simulink model "ACFT_cae"  (R2024a)
settings: Solver=ode4  StartTime=0.0  StopTime=10.0  FixedStep=0.01  RelTol=1e-3  EnableMultiTasking=on
values from neighbouring files (symbols this model uses):
  Inertia = [Ixx 0 0; 0 Iyy 0; 0 0 Izz]    [Initialization.m]    (also in Initialization_alt2.m; Initialization_cg1.m; Initialization_loop.m; Initialization_v2.m)
libraries: AerodynamicModel x1, AtmosphericModel x1, EqM x1, Propulsion x1
settings Model: Creator=Caê  LastModifiedBy=Caê
settings RTWCC: GPUComputeCapability=3.5

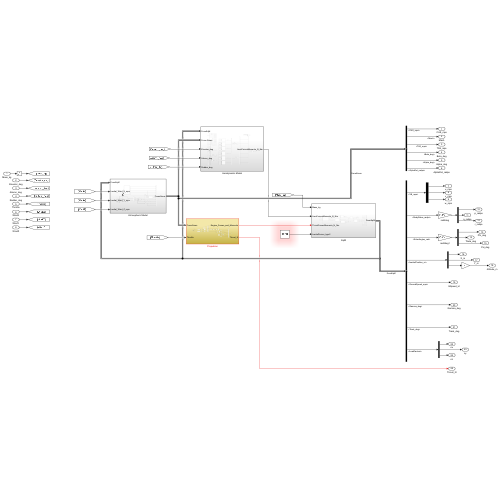
[thumbnail: Simulink's stored preview of the top-level diagram]
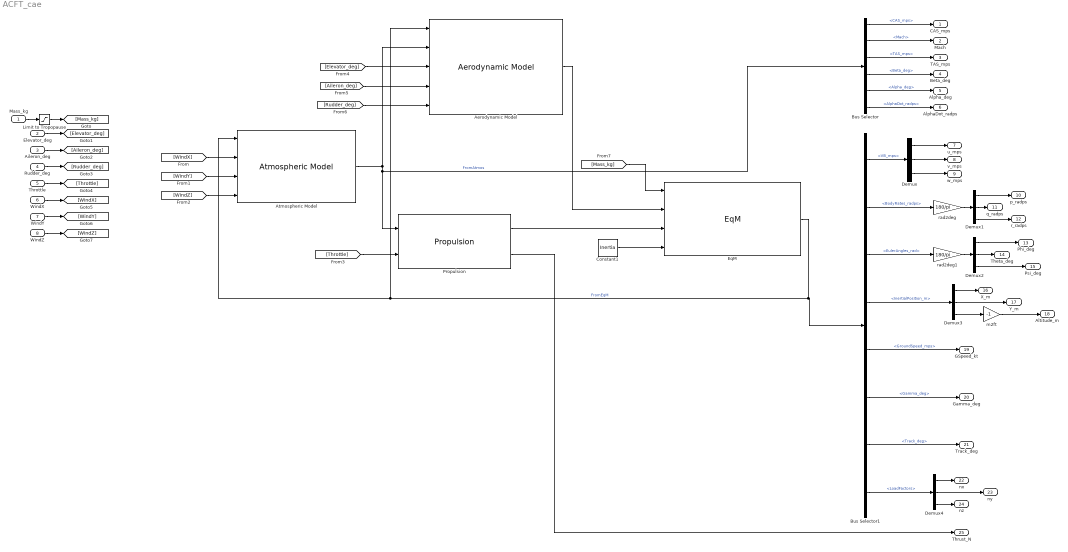
== system ACFT_cae ==
  Mass_kg : Inport
  Elevator_deg : Inport  Port=2
  Aileron_deg : Inport  Port=3
  Rudder_deg : Inport  Port=4
  Throttle : Inport  Port=5
  WindX : Inport  Port=6
  WindY : Inport  Port=7
  WindZ : Inport  Port=8
  Aerodynamic Model : AerodynamicModel/Aerodynamic Model  SystemSampleTime=-1  VariantActivationTime=update diagram  AllowFlexibleInterface=on  Latency=0  AutoFrameSizeCalculation=off
  Atmospheric Model : AtmosphericModel/Atmospheric Model  SystemSampleTime=-1  VariantActivationTime=update diagram  AllowFlexibleInterface=on  Latency=0  AutoFrameSizeCalculation=off
  Bus Selector : BusSelector  OutputSignals=CAS_mps,Mach,TAS_mps,Beta_deg,Alpha_deg,AlphaDot_radps
  Bus Selector1 : BusSelector  OutputSignals=VB_mps,BodyRates_radps,EulerAngles_rad,InertialPosition_m,GroundSpeed_mps,Gamma_deg,Track_deg,LoadFactors
  Constant1 : Constant  Value=Inertia
  Demux{,1..4} (5 alike) : Demux  Outputs=3
  EqM : EqM/EqM  SystemSampleTime=-1  VariantActivationTime=update diagram  AllowFlexibleInterface=on  Latency=0  AutoFrameSizeCalculation=off
  Limit to Tropopause : Saturate  UpperLimit=inf  LowerLimit=0.01
  Propulsion : Propulsion/Propulsion  SystemSampleTime=-1  VariantActivationTime=update diagram  AllowFlexibleInterface=on  Latency=0  AutoFrameSizeCalculation=off
  m2ft : Gain  Gain=-1
  rad2deg : Gain  Gain=180/pi
  rad2deg1 : Gain  Gain=180/pi
  CAS_mps : Outport
  Mach : Outport  Port=2
  TAS_mps : Outport  Port=3
  Beta_deg : Outport  Port=4
  Alpha_deg : Outport  Port=5
  AlphaDot_radps : Outport  Port=6
  u_mps : Outport  Port=7
  v_mps : Outport  Port=8
  w_mps : Outport  Port=9
  p_radps : Outport  Port=10
  q_radps : Outport  Port=11
  r_radps : Outport  Port=12
  Phi_deg : Outport  Port=13
  Theta_deg : Outport  Port=14
  Psi_deg : Outport  Port=15
  X_m : Outport  Port=16
  Y_m : Outport  Port=17
  Altitude_m : Outport  Port=18
  GSpeed_kt : Outport  Port=19
  Gamma_deg : Outport  Port=20
  Track_deg : Outport  Port=21
  nx : Outport  Port=22
  ny : Outport  Port=23
  nz : Outport  Port=24
  Thrust_N : Outport  Port=25
  wires:
  Atmospheric Model/1 -> Aerodynamic Model/2, Propulsion/1, Bus Selector/1  "FromAtmos"
  Propulsion/1 -> EqM/3
  Aerodynamic Model/1 -> EqM/2
  EqM/1 -> Bus Selector1/1, Atmospheric Model/1, Aerodynamic Model/1  "FromEqM"
  Constant1/1 -> EqM/4
  Mass_kg/1 -> Limit to Tropopause/1
  Elevator_deg/1 -> [Elevator_deg]
  Aileron_deg/1 -> [Aileron_deg]
  Rudder_deg/1 -> [Rudder_deg]
  Throttle/1 -> [Throttle]
  WindX/1 -> [WindX]
  WindY/1 -> [WindY]
  WindZ/1 -> [WindZ]
  [WindZ] -> Atmospheric Model/4
  [WindY] -> Atmospheric Model/3
  [WindX] -> Atmospheric Model/2
  [Throttle] -> Propulsion/2
  [Rudder_deg] -> Aerodynamic Model/5
  [Aileron_deg] -> Aerodynamic Model/4
  [Elevator_deg] -> Aerodynamic Model/3
  [Mass_kg] -> EqM/1
  Propulsion/2 -> Thrust_N/1
  Bus Selector/1 -> CAS_mps/1  "<CAS_mps>"
  Bus Selector/2 -> Mach/1  "<Mach>"
  Bus Selector/3 -> TAS_mps/1  "<TAS_mps>"
  Bus Selector/4 -> Beta_deg/1  "<Beta_deg>"
  Bus Selector/5 -> Alpha_deg/1  "<Alpha_deg>"
  Bus Selector/6 -> AlphaDot_radps/1  "<AlphaDot_radps>"
  Bus Selector1/1 -> Demux/1  "<VB_mps>"
  Demux/1 -> u_mps/1
  Demux/2 -> v_mps/1
  Demux/3 -> w_mps/1
  Demux1/3 -> r_radps/1
  Demux1/1 -> p_radps/1
  Demux1/2 -> q_radps/1
  Bus Selector1/2 -> rad2deg/1  "<BodyRates_radps>"
  Demux2/3 -> Psi_deg/1
  Demux2/1 -> Phi_deg/1
  Demux2/2 -> Theta_deg/1
  Bus Selector1/3 -> rad2deg1/1  "<EulerAngles_rad>"
  rad2deg/1 -> Demux1/1
  rad2deg1/1 -> Demux2/1
  Bus Selector1/4 -> Demux3/1  "<InertialPosition_m>"
  Demux3/1 -> X_m/1
  Demux3/2 -> Y_m/1
  Demux3/3 -> m2ft/1
  m2ft/1 -> Altitude_m/1
  Bus Selector1/5 -> GSpeed_kt/1  "<GroundSpeed_mps>"
  Bus Selector1/6 -> Gamma_deg/1  "<Gamma_deg>"
  Bus Selector1/7 -> Track_deg/1  "<Track_deg>"
  Bus Selector1/8 -> Demux4/1  "<LoadFactors>"
  Demux4/3 -> nz/1
  Demux4/2 -> ny/1
  Demux4/1 -> nx/1
  Limit to Tropopause/1 -> [Mass_kg]
